simulink model "CL_LQG_2021a"  (R2021a)
settings: Solver=ode15s  StartTime=0.0  StopTime=1250  RelTol=1e-3
values from neighbouring files (symbols this model uses):
  A_kf = [-0.0171366511824 0.0171366511824 0 0 -0.405989384527 -1.0114279511 -4.63493813994e-17 -1.85727570483e-16 0 0 -0.052376732387 0.052376732387 ... (16 elements, 4x4)]    [parameters.mat]
  B_kf = [0 0.120715699163 0.138722651778 0 0.0970102697521 0 0 0.159450121706 0.405989384527 0.916181411394 4.63493813994e-17 1.85727570483e-16 ... (16 elements, 4x4)]    [parameters.mat]
  C = [   0,      1,      0,      0 ... (first row only)    [linearize_4tanks.m]    (also in parameters.mat = [0  1  0  0; 0  0  0  1])
  C_kf = [1 0 0 0 0 1 0 0 0 0 1 0 ... (16 elements, 4x4)]    [parameters.mat]
  D_kf = [0 0 0 0 0 0 0 0 0 0 0 0 ... (16 elements, 4x4)]    [parameters.mat]
  K_integrators = [-0.0995479981451  -0.00949716090787; 0.00949716090787  -0.0995479981451]    [parameters.mat]
  K_state = [0.12950650673  0.722856465098  0.0139705767535  0.0637209208421; -0.0211766819284  -0.0833619871599  0.236348353203  0.657206774714]    [parameters.mat]
  u_bar = reshape(z_opt(5:6), [2, 1])    [linearize_4tanks.m]    (also in parameters.mat = [6.60003195923 9.28189672086])
  x_bar = reshape(z_opt(1:4), [4, 1])    [linearize_4tanks.m]    (also in parameters.mat = [24.6597369405 10 3.03378366821 10])
undefined symbols (not defined in the file or in its folder): AA, h0, xv, ygamma1, ygamma2, yk1, yk2
libraries: simulink x4, simulink_extras x4
settings Model: Creator=fabio  LastModifiedBy=ermarinellone
settings OptimizationCC: BlockReduction=off  DefaultParameterBehavior=Inlined  BufferReuse=off
settings DebuggingCC: UnconnectedInputMsg=none  UnconnectedOutputMsg=none  UnconnectedLineMsg=none
settings ModelReferenceCC: EnableRefExpFcnMdlSchedulingChecks=off
settings RTWCC: Description=Generic Real-Time Target  DLArmComputeVersion=20.02.1

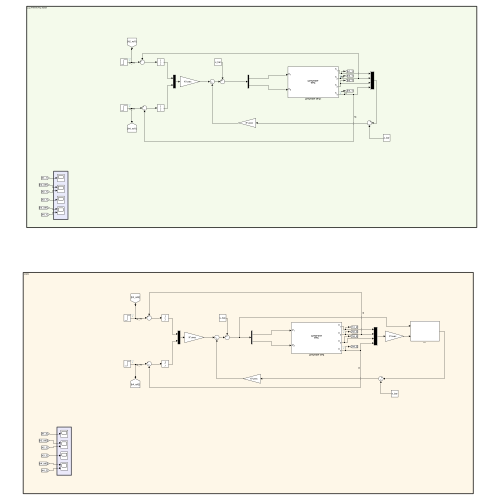
[thumbnail: Simulink's stored preview of the top-level diagram]
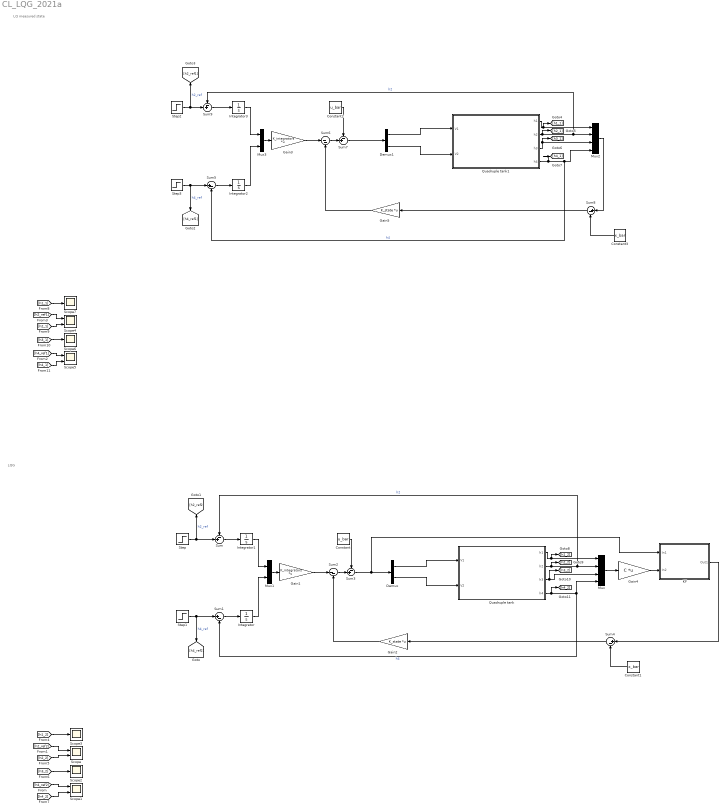
== system CL_LQG_2021a ==
  note: LQG
  note: LQ measured state
  Constant : Constant  Value=u_bar
  Constant1 : Constant  Value=x_bar
  Constant2 : Constant  Value=u_bar
  Constant3 : Constant  Value=x_bar
  Demux : Demux  Outputs=2
  Demux1 : Demux  Outputs=2
  Gain1 : Gain  Gain=K_integrators  Multiplication=Matrix(K*u) (u vector)
  Gain2 : Gain  Gain=K_state  Multiplication=Matrix(K*u) (u vector)
  Gain3 : Gain  Gain=K_integrators  Multiplication=Matrix(K*u) (u vector)
  Gain4 : Gain  Gain=C  Multiplication=Matrix(K*u) (u vector)
  Gain5 : Gain  Gain=K_state  Multiplication=Matrix(K*u) (u vector)
  Integrator{,1..3} (4 alike) : Integrator
  KF : Subsystem
  Mux : Mux
  Mux1 : Mux  Inputs=2
  Mux2 : Mux
  Mux3 : Mux  Inputs=2
  Quadruple tank : Subsystem  mask{h_0=h0, A=AA, S=(4.44 / 2)^2 * pi * ones(1, 4), g=981}
      mask prompts: h_0 "Initial level"; A "Outlet section"; S "Tank section"; g "Gravity"
      mask DialogControl h_0 Tooltip: [cm]
      mask DialogControl A Tooltip: [cm^2]
      mask DialogControl S Tooltip: [cm^2]
      mask DialogControl g Tooltip: [cm/s^2]
      mask Display:
      | disp('Quadruple\nTank');
      | port_label('input', 1, 'V_1', 'interpreter', 'tex');
      | port_label('input', 2, 'V_2', 'interpreter', 'tex');
      | port_label('output', 1, 'h_1', 'interpreter', 'tex');
      | port_label('output', 2, 'h_2', 'interpreter', 'tex');
      | port_label('output', 3, 'h_3', 'interpreter', 'tex');
      | port_label('output', 4, 'h_4', 'interpreter', 'tex');
  Quadruple tank1 : Subsystem  mask{h_0=h0, A=AA, S=(4.44 / 2)^2 * pi * ones(1, 4), g=981}
      mask prompts: h_0 "Initial level"; A "Outlet section"; S "Tank section"; g "Gravity"
      mask DialogControl h_0 Tooltip: [cm]
      mask DialogControl A Tooltip: [cm^2]
      mask DialogControl S Tooltip: [cm^2]
      mask DialogControl g Tooltip: [cm/s^2]
      mask Display:
      | disp('Quadruple\nTank');
      | port_label('input', 1, 'V_1', 'interpreter', 'tex');
      | port_label('input', 2, 'V_2', 'interpreter', 'tex');
      | port_label('output', 1, 'h_1', 'interpreter', 'tex');
      | port_label('output', 2, 'h_2', 'interpreter', 'tex');
      | port_label('output', 3, 'h_3', 'interpreter', 'tex');
      | port_label('output', 4, 'h_4', 'interpreter', 'tex');
  Scope{,1,4..5} (4 alike) : Scope  NumInputPorts=2
  Scope{2..3,6..7} (4 alike) : Scope
  Step : Step  Time=500  Before=10  After=13  SampleTime=0
  Step1 : Step  Time=500  Before=10  After=10  SampleTime=0
  Step2 : Step  Time=500  Before=10  After=13  SampleTime=0
  Step3 : Step  Time=500  Before=10  After=10  SampleTime=0
  Sum{,3,7,9} (4 alike) : Sum  Inputs=-+|
  Sum{1,4..5,8} (4 alike) : Sum  Inputs=|+-
  Sum2 : Sum  Inputs=|--
  Sum6 : Sum  Inputs=|--
  wires:
  Step/1 -> Sum/2, [h2_ref2]  "h2_ref"
  Quadruple tank/2(h2) -> [h2_2], Sum/1, Mux/2  "h2"
  Quadruple tank/1(h1) -> [h1_2], Mux/1
  Quadruple tank/3(h3) -> [h3_2], Mux/3
  Quadruple tank/4(h4) -> [h4_2], Sum1/2, Mux/4  "h4"
  Step1/1 -> Sum1/1, [h4_ref2]  "h4_ref"
  [h4_ref2] -> Scope1/1
  [h2_ref2] -> Scope/1
  Sum/1 -> Integrator1/1
  Sum1/1 -> Integrator/1
  Integrator1/1 -> Mux1/1
  Integrator/1 -> Mux1/2
  Constant/1 -> Sum3/1
  Sum2/1 -> Sum3/2
  Mux1/1 -> Gain1/1
  Gain1/1 -> Sum2/1
  Gain2/1 -> Sum2/2
  Sum3/1 -> KF/1(In1), Demux/1
  Demux/1 -> Quadruple tank/1(V1)
  Demux/2 -> Quadruple tank/2(V2)
  Mux/1 -> Gain4/1
  Gain4/1 -> KF/2(In2)
  Sum4/1 -> Gain2/1
  Constant1/1 -> Sum4/2
  Quadruple tank1/2(h2) -> [h2_1], Mux2/2, Sum9/1  "h2"
  Quadruple tank1/1(h1) -> [h1_1], Mux2/1
  Quadruple tank1/3(h3) -> Mux2/3, [h3_1]
  Demux1/1 -> Quadruple tank1/1(V1)
  Step3/1 -> Sum5/1, [h4_ref1]  "h4_ref"
  Step2/1 -> Sum9/2, [h2_ref1]  "h2_ref"
  Demux1/2 -> Quadruple tank1/2(V2)
  [h1_2] -> Scope3/1
  [h2_2] -> Scope/2
  [h3_2] -> Scope2/1
  [h4_2] -> Scope1/2
  [h1_1] -> Scope7/1
  [h2_ref1] -> Scope4/1
  [h2_1] -> Scope4/2
  [h3_1] -> Scope6/1
  [h4_ref1] -> Scope5/1
  [h4_1] -> Scope5/2
  Constant3/1 -> Sum8/2
  Integrator3/1 -> Mux3/1
  Sum9/1 -> Integrator3/1
  Sum7/1 -> Demux1/1
  Quadruple tank1/4(h4) -> [h4_1], Sum5/2, Mux2/4  "h4"
  Integrator2/1 -> Mux3/2
  Sum6/1 -> Sum7/2
  Mux2/1 -> Sum8/1
  Mux3/1 -> Gain3/1
  Gain5/1 -> Sum6/2
  Gain3/1 -> Sum6/1
  Sum8/1 -> Gain5/1
  Constant2/1 -> Sum7/1
  Sum5/1 -> Integrator2/1
  KF/1(Out1) -> Sum4/1

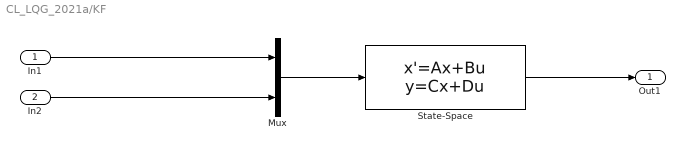
== system CL_LQG_2021a/KF ==
  In1 : Inport
  In2 : Inport  Port=2
  Mux : Mux  Inputs=2
  State-Space : StateSpace  A=A_kf  B=B_kf  C=C_kf  D=D_kf  InitialCondition=0
  Out1 : Outport
  wires:
  In1/1 -> Mux/1
  Mux/1 -> State-Space/1
  State-Space/1 -> Out1/1
  In2/1 -> Mux/2

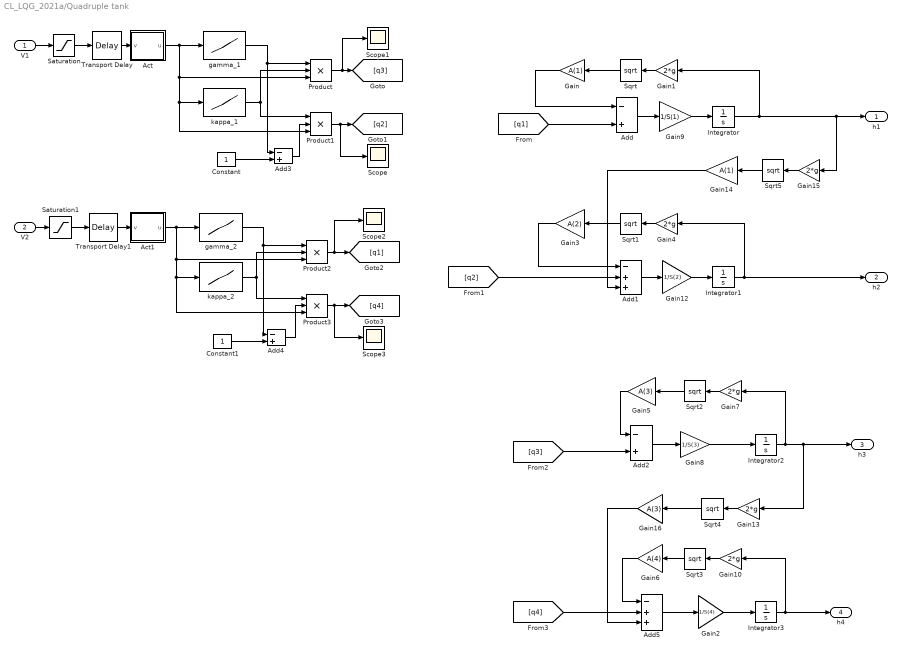
== system CL_LQG_2021a/Quadruple tank ==
  V1 : Inport
  V2 : Inport  Port=2
  Act : Subsystem
  Act1 : Subsystem
  Add{,2..4} (4 alike) : Sum  Inputs=-+
  Add1 : Sum  Inputs=-++
  Add5 : Sum  Inputs=-++
  Constant : Constant
  Constant1 : Constant
  Gain : Gain  Gain=A(1)
  Gain{1,4,7,10,13,15} (6 alike) : Gain  Gain=2*g
  Gain12 : Gain  Gain=1/S(2)
  Gain14 : Gain  Gain=A(1)
  Gain16 : Gain  Gain=A(3)
  Gain2 : Gain  Gain=1/S(4)
  Gain3 : Gain  Gain=A(2)
  Gain5 : Gain  Gain=A(3)
  Gain6 : Gain  Gain=A(4)
  Gain8 : Gain  Gain=1/S(3)
  Gain9 : Gain  Gain=1/S(1)
  Integrator : Integrator  InitialCondition=h_0(1)  LimitOutput=on  UpperSaturationLimit=30  LowerSaturationLimit=0
  Integrator1 : Integrator  InitialCondition=h_0(2)  LimitOutput=on  UpperSaturationLimit=30  LowerSaturationLimit=0
  Integrator2 : Integrator  InitialCondition=h_0(3)  LimitOutput=on  UpperSaturationLimit=30  LowerSaturationLimit=0
  Integrator3 : Integrator  InitialCondition=h_0(4)  LimitOutput=on  UpperSaturationLimit=30  LowerSaturationLimit=0
  Product{,1..3} (4 alike) : Product  Inputs=3
  Saturation : Saturate  UpperLimit=18  LowerLimit=0
  Saturation1 : Saturate  UpperLimit=18  LowerLimit=0
  Scope{,1..3} (4 alike) : Scope
  Sqrt{,1..5} (6 alike) : Sqrt  SaturateOnIntegerOverflow=on
  Transport Delay : TransportDelay  DelayTime=2
  Transport Delay1 : TransportDelay  DelayTime=2
  gamma_1 : Lookup_n-D  NumberOfTableDimensions=1  BreakpointsForDimension1=xv  Table=ygamma1  ExtrapMethod=Clip  UseLastTableValue=on  InternalRulePriority=Speed  RndMeth=Simplest  InputSameDT=on
  gamma_2 : Lookup_n-D  NumberOfTableDimensions=1  BreakpointsForDimension1=xv  Table=ygamma2  ExtrapMethod=Clip  UseLastTableValue=on  InternalRulePriority=Speed  RndMeth=Simplest  InputSameDT=on
  kappa_1 : Lookup_n-D  NumberOfTableDimensions=1  BreakpointsForDimension1=xv  Table=yk1  ExtrapMethod=Clip  UseLastTableValue=on  InternalRulePriority=Speed  RndMeth=Simplest  InputSameDT=on
  kappa_2 : Lookup_n-D  NumberOfTableDimensions=1  BreakpointsForDimension1=xv  Table=yk2  ExtrapMethod=Clip  UseLastTableValue=on  InternalRulePriority=Speed  RndMeth=Simplest  InputSameDT=on
  h1 : Outport
  h2 : Outport  Port=2
  h3 : Outport  Port=3
  h4 : Outport  Port=4
  wires:
  Integrator/1 -> Gain15/1, h1/1, Gain1/1
  Gain1/1 -> Sqrt/1
  Sqrt/1 -> Gain/1
  Gain/1 -> Add/1
  [q1] -> Add/2
  Add1/1 -> Gain12/1
  Integrator1/1 -> Gain4/1, h2/1
  Gain4/1 -> Sqrt1/1
  Add2/1 -> Gain8/1
  Gain7/1 -> Sqrt2/1
  Sqrt2/1 -> Gain5/1
  Gain6/1 -> Add5/1
  Sqrt3/1 -> Gain6/1
  Gain10/1 -> Sqrt3/1
  Integrator3/1 -> Gain10/1, h4/1
  [q4] -> Add5/2
  Sqrt4/1 -> Gain16/1
  Gain13/1 -> Sqrt4/1
  Integrator2/1 -> Gain7/1, h3/1, Gain13/1
  Sqrt1/1 -> Gain3/1
  Gain3/1 -> Add1/1
  Gain5/1 -> Add2/1
  Gain15/1 -> Sqrt5/1
  Sqrt5/1 -> Gain14/1
  Gain14/1 -> Add1/3
  [q2] -> Add1/2
  [q3] -> Add2/2
  Gain16/1 -> Add5/3
  gamma_1/1 -> Add3/1, Product/1
  Constant/1 -> Add3/2
  kappa_1/1 -> Product/2, Product1/1
  Add3/1 -> Product1/2
  Product/1 -> Scope1/1, [q3]
  Product1/1 -> Scope/1, [q2]
  kappa_2/1 -> Product3/1, Product2/2
  Product2/1 -> Scope2/1, [q1]
  Constant1/1 -> Add4/2
  gamma_2/1 -> Add4/1, Product2/1
  Product3/1 -> Scope3/1, [q4]
  Add4/1 -> Product3/2
  Gain12/1 -> Integrator1/1
  Add/1 -> Gain9/1
  Gain9/1 -> Integrator/1
  Gain8/1 -> Integrator2/1
  Add5/1 -> Gain2/1
  Gain2/1 -> Integrator3/1
  Act/1(u) -> gamma_1/1, Product/3, kappa_1/1, Product1/3
  Act1/1(u) -> gamma_2/1, Product2/3, kappa_2/1, Product3/3
  Transport Delay/1 -> Act/1(v)
  V1/1 -> Saturation/1
  Saturation/1 -> Transport Delay/1
  Saturation1/1 -> Transport Delay1/1
  V2/1 -> Saturation1/1
  Transport Delay1/1 -> Act1/1(v)

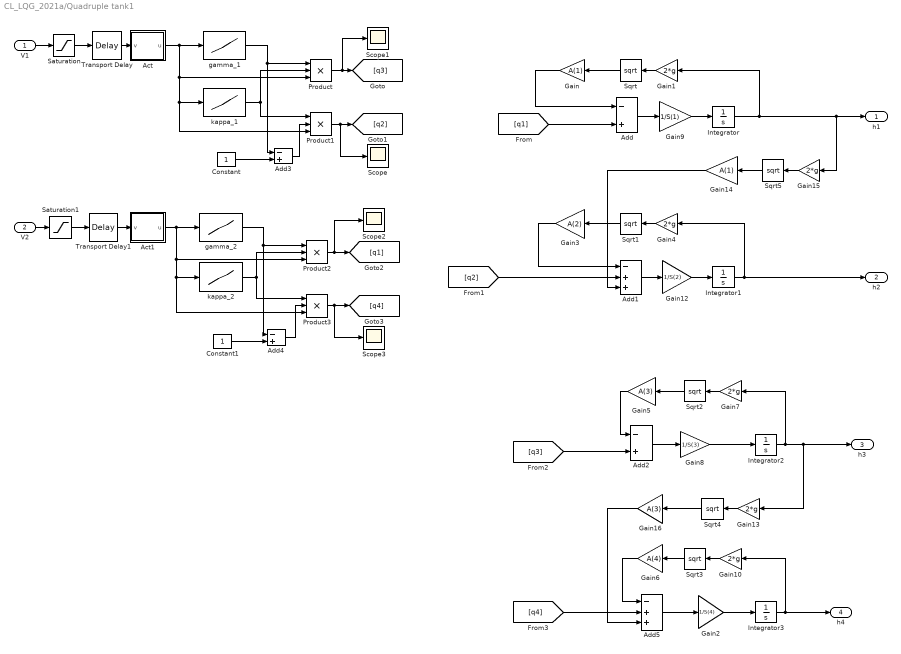
== system CL_LQG_2021a/Quadruple tank1 ==
  V1 : Inport
  V2 : Inport  Port=2
  Act : Subsystem
  Act1 : Subsystem
  Add{,2..4} (4 alike) : Sum  Inputs=-+
  Add1 : Sum  Inputs=-++
  Add5 : Sum  Inputs=-++
  Constant : Constant
  Constant1 : Constant
  Gain : Gain  Gain=A(1)
  Gain{1,4,7,10,13,15} (6 alike) : Gain  Gain=2*g
  Gain12 : Gain  Gain=1/S(2)
  Gain14 : Gain  Gain=A(1)
  Gain16 : Gain  Gain=A(3)
  Gain2 : Gain  Gain=1/S(4)
  Gain3 : Gain  Gain=A(2)
  Gain5 : Gain  Gain=A(3)
  Gain6 : Gain  Gain=A(4)
  Gain8 : Gain  Gain=1/S(3)
  Gain9 : Gain  Gain=1/S(1)
  Integrator : Integrator  InitialCondition=h_0(1)  LimitOutput=on  UpperSaturationLimit=30  LowerSaturationLimit=0
  Integrator1 : Integrator  InitialCondition=h_0(2)  LimitOutput=on  UpperSaturationLimit=30  LowerSaturationLimit=0
  Integrator2 : Integrator  InitialCondition=h_0(3)  LimitOutput=on  UpperSaturationLimit=30  LowerSaturationLimit=0
  Integrator3 : Integrator  InitialCondition=h_0(4)  LimitOutput=on  UpperSaturationLimit=30  LowerSaturationLimit=0
  Product{,1..3} (4 alike) : Product  Inputs=3
  Saturation : Saturate  UpperLimit=18  LowerLimit=0
  Saturation1 : Saturate  UpperLimit=18  LowerLimit=0
  Scope{,1..3} (4 alike) : Scope
  Sqrt{,1..5} (6 alike) : Sqrt  SaturateOnIntegerOverflow=on
  Transport Delay : TransportDelay  DelayTime=2
  Transport Delay1 : TransportDelay  DelayTime=2
  gamma_1 : Lookup_n-D  NumberOfTableDimensions=1  BreakpointsForDimension1=xv  Table=ygamma1  ExtrapMethod=Clip  UseLastTableValue=on  InternalRulePriority=Speed  RndMeth=Simplest  InputSameDT=on
  gamma_2 : Lookup_n-D  NumberOfTableDimensions=1  BreakpointsForDimension1=xv  Table=ygamma2  ExtrapMethod=Clip  UseLastTableValue=on  InternalRulePriority=Speed  RndMeth=Simplest  InputSameDT=on
  kappa_1 : Lookup_n-D  NumberOfTableDimensions=1  BreakpointsForDimension1=xv  Table=yk1  ExtrapMethod=Clip  UseLastTableValue=on  InternalRulePriority=Speed  RndMeth=Simplest  InputSameDT=on
  kappa_2 : Lookup_n-D  NumberOfTableDimensions=1  BreakpointsForDimension1=xv  Table=yk2  ExtrapMethod=Clip  UseLastTableValue=on  InternalRulePriority=Speed  RndMeth=Simplest  InputSameDT=on
  h1 : Outport
  h2 : Outport  Port=2
  h3 : Outport  Port=3
  h4 : Outport  Port=4
  wires:
  Integrator/1 -> Gain15/1, h1/1, Gain1/1
  Gain1/1 -> Sqrt/1
  Sqrt/1 -> Gain/1
  Gain/1 -> Add/1
  [q1] -> Add/2
  Add1/1 -> Gain12/1
  Integrator1/1 -> Gain4/1, h2/1
  Gain4/1 -> Sqrt1/1
  Add2/1 -> Gain8/1
  Gain7/1 -> Sqrt2/1
  Sqrt2/1 -> Gain5/1
  Gain6/1 -> Add5/1
  Sqrt3/1 -> Gain6/1
  Gain10/1 -> Sqrt3/1
  Integrator3/1 -> Gain10/1, h4/1
  [q4] -> Add5/2
  Sqrt4/1 -> Gain16/1
  Gain13/1 -> Sqrt4/1
  Integrator2/1 -> Gain7/1, h3/1, Gain13/1
  Sqrt1/1 -> Gain3/1
  Gain3/1 -> Add1/1
  Gain5/1 -> Add2/1
  Gain15/1 -> Sqrt5/1
  Sqrt5/1 -> Gain14/1
  Gain14/1 -> Add1/3
  [q2] -> Add1/2
  [q3] -> Add2/2
  Gain16/1 -> Add5/3
  gamma_1/1 -> Add3/1, Product/1
  Constant/1 -> Add3/2
  kappa_1/1 -> Product/2, Product1/1
  Add3/1 -> Product1/2
  Product/1 -> Scope1/1, [q3]
  Product1/1 -> Scope/1, [q2]
  kappa_2/1 -> Product3/1, Product2/2
  Product2/1 -> Scope2/1, [q1]
  Constant1/1 -> Add4/2
  gamma_2/1 -> Add4/1, Product2/1
  Product3/1 -> Scope3/1, [q4]
  Add4/1 -> Product3/2
  Gain12/1 -> Integrator1/1
  Add/1 -> Gain9/1
  Gain9/1 -> Integrator/1
  Gain8/1 -> Integrator2/1
  Add5/1 -> Gain2/1
  Gain2/1 -> Integrator3/1
  Act/1(u) -> gamma_1/1, Product/3, kappa_1/1, Product1/3
  Act1/1(u) -> gamma_2/1, Product2/3, kappa_2/1, Product3/3
  Transport Delay/1 -> Act/1(v)
  V1/1 -> Saturation/1
  Saturation/1 -> Transport Delay/1
  Saturation1/1 -> Transport Delay1/1
  V2/1 -> Saturation1/1
  Transport Delay1/1 -> Act1/1(v)

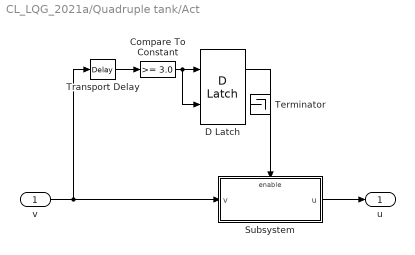
== system CL_LQG_2021a/Quadruple tank/Act ==
  v : Inport
  Compare To Constant : simulink/Logic and Bit Operations/Compare To Constant  relop=>=  const=3.0  OutDataTypeStr=boolean
  D Latch : simulink_extras/Flip Flops/D Latch
  Subsystem : Subsystem
  Terminator : Terminator
  Transport Delay : TransportDelay  DelayTime=4
  u : Outport
  wires:
  v/1 -> Transport Delay/1, Subsystem/1(v)
  D Latch/1 -> Subsystem/Enable
  Subsystem/1(u) -> u/1
  Transport Delay/1 -> Compare To Constant/1
  Compare To Constant/1 -> D Latch/2, D Latch/1

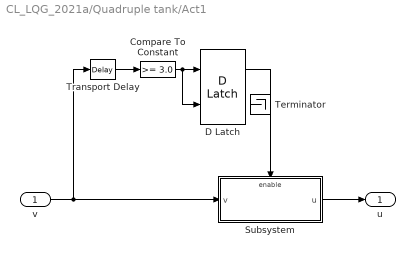
== system CL_LQG_2021a/Quadruple tank/Act1 ==
  v : Inport
  Compare To Constant : simulink/Logic and Bit Operations/Compare To Constant  relop=>=  const=3.0  OutDataTypeStr=boolean
  D Latch : simulink_extras/Flip Flops/D Latch
  Subsystem : Subsystem
  Terminator : Terminator
  Transport Delay : TransportDelay  DelayTime=4
  u : Outport
  wires:
  v/1 -> Transport Delay/1, Subsystem/1(v)
  D Latch/1 -> Subsystem/Enable
  Subsystem/1(u) -> u/1
  Transport Delay/1 -> Compare To Constant/1
  Compare To Constant/1 -> D Latch/2, D Latch/1

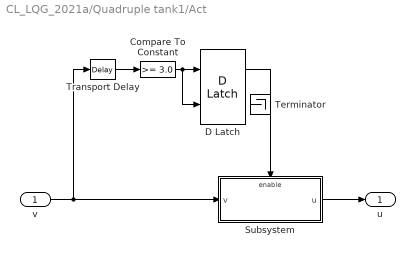
== system CL_LQG_2021a/Quadruple tank1/Act ==
  v : Inport
  Compare To Constant : simulink/Logic and Bit Operations/Compare To Constant  relop=>=  const=3.0  OutDataTypeStr=boolean
  D Latch : simulink_extras/Flip Flops/D Latch
  Subsystem : Subsystem
  Terminator : Terminator
  Transport Delay : TransportDelay  DelayTime=4
  u : Outport
  wires:
  v/1 -> Transport Delay/1, Subsystem/1(v)
  D Latch/1 -> Subsystem/Enable
  Subsystem/1(u) -> u/1
  Transport Delay/1 -> Compare To Constant/1
  Compare To Constant/1 -> D Latch/2, D Latch/1

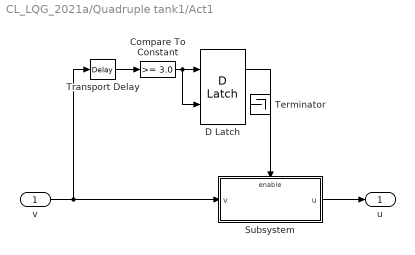
== system CL_LQG_2021a/Quadruple tank1/Act1 ==
  v : Inport
  Compare To Constant : simulink/Logic and Bit Operations/Compare To Constant  relop=>=  const=3.0  OutDataTypeStr=boolean
  D Latch : simulink_extras/Flip Flops/D Latch
  Subsystem : Subsystem
  Terminator : Terminator
  Transport Delay : TransportDelay  DelayTime=4
  u : Outport
  wires:
  v/1 -> Transport Delay/1, Subsystem/1(v)
  D Latch/1 -> Subsystem/Enable
  Subsystem/1(u) -> u/1
  Transport Delay/1 -> Compare To Constant/1
  Compare To Constant/1 -> D Latch/2, D Latch/1

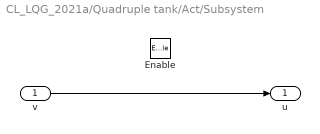
== system CL_LQG_2021a/Quadruple tank/Act/Subsystem ==
  v : Inport
  Enable : EnablePort
  u : Outport
  wires:
  v/1 -> u/1

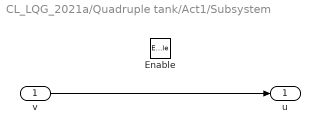
== system CL_LQG_2021a/Quadruple tank/Act1/Subsystem ==
  v : Inport
  Enable : EnablePort
  u : Outport
  wires:
  v/1 -> u/1

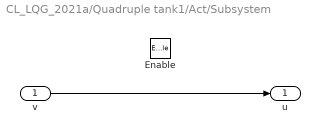
== system CL_LQG_2021a/Quadruple tank1/Act/Subsystem ==
  v : Inport
  Enable : EnablePort
  u : Outport
  wires:
  v/1 -> u/1

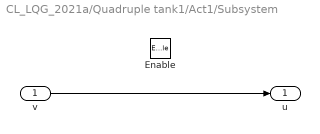
== system CL_LQG_2021a/Quadruple tank1/Act1/Subsystem ==
  v : Inport
  Enable : EnablePort
  u : Outport
  wires:
  v/1 -> u/1
